simulink model "NE39bus_modified"  (R2025b)
settings: Solver=ode23tb  StartTime=0.0  StopTime=10  MaxStep=0.001  RelTol=1e-4  AbsTol=1e-6  EnableMultiTasking=on
PreLoadFcn:
  | NE39bus_data;
  | PSSMODEL=1;
  | LPSS=0;
  | WAPSS=0;
  | WAPSS2=0;
model workspace (MAT data in the model file):
  DT = 0.2
  T_EPISODE = 10
  VSG_D0 = 3
  VSG_M0 = 12
  omega_n = 314.159265359
values from neighbouring files (symbols this model uses):
  AVR_Data = [     0.01  200    0.015   10    1    1.03    -5    5 ... (first row only)    [NE39bus_data.m]    (also in NE39bus_workspace.mat = [0.01 0.01 0.01 0.01 0.01 0.01 0.01 0.01 0.01 0.01 200 200 .)
  line = [     1	2	0.0035	0.0411	0.6987	0	100	345 ... (first row only)    [NE39bus_data.m]    (also in NE39bus_modified_data.m = [     1   2   0.0035  0.0411  0.6987  0   100 345; NE39bus_workspace.mat = [1 1 2 2 2 3 3 4 4 5 6 6 ... (368 elements, 46x8)])
  mac_con = [ ... (first row only)    [NE39bus_data.m]    (also in NE39bus_workspace.mat = [1 2 3 4 5 6 7 8 9 10 39 31 ... (190 elements, 10x19)])
  MB = [1   0.2 30   1.25 40    12 160]    [NE39bus_data.m]    (also in NE39bus_modified_data.m = [1  0.2  30  1.25  40  12  160]; NE39bus_workspace.mat = [1 0.2 30 1.25 40 12 160])
  Ns = 120*60/(2)    (= 3600)    [NE39bus_data.m]    (also in NE39bus_workspace.mat)
  p0 = [1000 520.81 650 632 508 650 560 540 830 250]'./1000    [NE39bus_data.m]    (also in NE39bus_workspace.mat = [1 0.52081 0.65 0.632 0.508 0.65 0.56 0.54 0.83 0.25])
  Pn = [1 1 1 1 1 1 1 1 1 1]    [NE39bus_workspace.mat]
  s = 10    [NE39bus_data.m]    (also in NE39bus_workspace.mat)
undefined symbols (not defined in the file or in its folder): D1, Delta
libraries: spsThreePhaseVIMeasurementLib x48, spsThreePhasePISectionLineLib x34, spsGenericPowerSystemStabilizerLib x20, spsThreePhaseParallelRLCLoadLib x19, spsThreePhaseTransformerTwoWindingsLib x12, spsSynchronousMachinepuStandardLib x10, spsExcitationSystemLib x10, spsMultiBandPowerSystemStabilizerLib x10, spsSteamTurbineandGovernorLib x10, spsLoadFlowBusLib x10, spsThreePhaseProgrammableVoltageSourceLib x8, spsThreePhaseSeriesRLCBranchLib x8
(part 2 of 3)

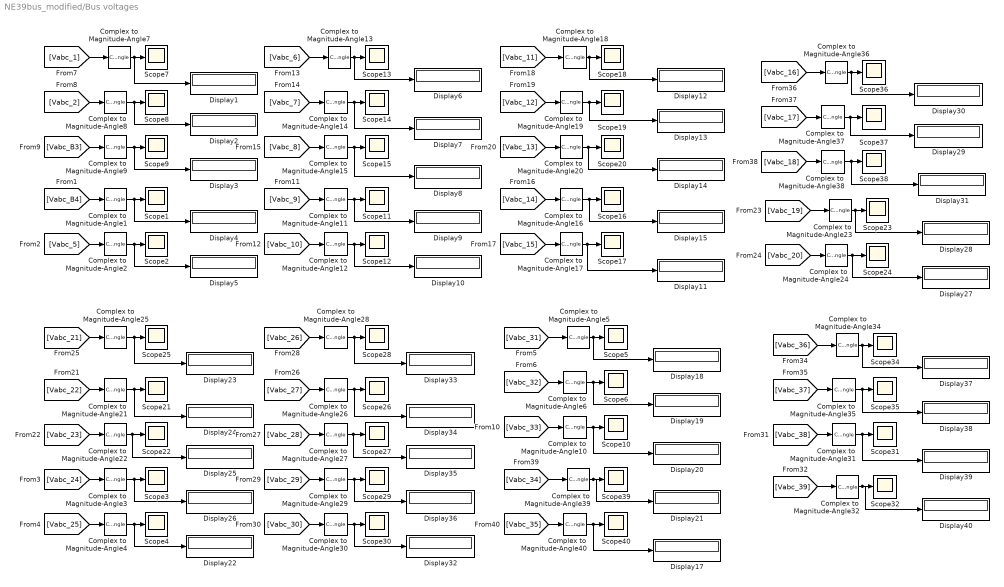
== system NE39bus_modified/Bus voltages ==
  Complex to Magnitude-Angle{1..32,34..40} (39 alike) : ComplexToMagnitudeAngle  Output=Magnitude
  Display{1..15,17..40} (39 alike) : Display
  Scope{1..32,34..40} (39 alike) : Scope
      Scope1 settings: ActiveDisplayYMinimum=-0.07  ActiveDisplayYMaximum=0.07  DataLoggingVariableName=v
      Scope10 settings: ActiveDisplayYMinimum=-0.07  ActiveDisplayYMaximum=0.07  DataLoggingVariableName=v2
      Scope11 settings: ActiveDisplayYMinimum=-0.07  ActiveDisplayYMaximum=0.07  DataLoggingVariableName=v11
      Scope12 settings: ActiveDisplayYMinimum=-0.07  ActiveDisplayYMaximum=0.07  DataLoggingVariableName=v12
      Scope13 settings: ActiveDisplayYMinimum=-0.07  ActiveDisplayYMaximum=0.07  DataLoggingVariableName=v13
      Scope14 settings: ActiveDisplayYMinimum=-0.07  ActiveDisplayYMaximum=0.07  DataLoggingVariableName=v14
      Scope15 settings: ActiveDisplayYMinimum=-0.07  ActiveDisplayYMaximum=0.07  DataLoggingVariableName=v15
      Scope16 settings: ActiveDisplayYMinimum=-0.07  ActiveDisplayYMaximum=0.07  DataLoggingVariableName=v16
      Scope17 settings: ActiveDisplayYMinimum=-0.07  ActiveDisplayYMaximum=0.07  DataLoggingVariableName=v17
      Scope18 settings: ActiveDisplayYMinimum=-0.07  ActiveDisplayYMaximum=0.07  DataLoggingVariableName=v18
      Scope19 settings: ActiveDisplayYMinimum=-0.07  ActiveDisplayYMaximum=0.07  DataLoggingVariableName=v19
      Scope2 settings: ActiveDisplayYMinimum=-0.07  ActiveDisplayYMaximum=0.07  DataLoggingVariableName=v1
      Scope20 settings: ActiveDisplayYMinimum=-0.07  ActiveDisplayYMaximum=0.07  DataLoggingVariableName=v20
      Scope21 settings: ActiveDisplayYMinimum=-0.07  ActiveDisplayYMaximum=0.07  DataLoggingVariableName=v21
      Scope22 settings: ActiveDisplayYMinimum=-0.07  ActiveDisplayYMaximum=0.07  DataLoggingVariableName=v22
      Scope23 settings: ActiveDisplayYMinimum=-0.07  ActiveDisplayYMaximum=0.07  DataLoggingVariableName=v68
      Scope24 settings: ActiveDisplayYMinimum=-0.07  ActiveDisplayYMaximum=0.07  DataLoggingVariableName=v69
      Scope25 settings: ActiveDisplayYMinimum=-0.07  ActiveDisplayYMaximum=0.07  DataLoggingVariableName=v70
      Scope26 settings: ActiveDisplayYMinimum=-0.07  ActiveDisplayYMaximum=0.07  DataLoggingVariableName=v63
      Scope27 settings: ActiveDisplayYMinimum=-0.07  ActiveDisplayYMaximum=0.07  DataLoggingVariableName=v64
      Scope28 settings: ActiveDisplayYMinimum=-0.07  ActiveDisplayYMaximum=0.07  DataLoggingVariableName=v65
      Scope29 settings: ActiveDisplayYMinimum=-0.07  ActiveDisplayYMaximum=0.07  DataLoggingVariableName=v66
      Scope3 settings: ActiveDisplayYMinimum=-0.07  ActiveDisplayYMaximum=0.07  DataLoggingVariableName=v3
      Scope30 settings: ActiveDisplayYMinimum=-0.07  ActiveDisplayYMaximum=0.07  DataLoggingVariableName=v67
      Scope31 settings: ActiveDisplayYMinimum=-0.07  ActiveDisplayYMaximum=0.07  DataLoggingVariableName=v71
      Scope32 settings: ActiveDisplayYMinimum=-0.07  ActiveDisplayYMaximum=0.07  DataLoggingVariableName=v72
      Scope34 settings: ActiveDisplayYMinimum=-0.07  ActiveDisplayYMaximum=0.07  DataLoggingVariableName=v74
      Scope35 settings: ActiveDisplayYMinimum=-0.07  ActiveDisplayYMaximum=0.07  DataLoggingVariableName=v75
      Scope36 settings: ActiveDisplayYMinimum=-0.07  ActiveDisplayYMaximum=0.07  DataLoggingVariableName=v48
      Scope37 settings: ActiveDisplayYMinimum=-0.07  ActiveDisplayYMaximum=0.07  DataLoggingVariableName=v49
      Scope38 settings: ActiveDisplayYMinimum=-0.07  ActiveDisplayYMaximum=0.07  DataLoggingVariableName=v50
      Scope39 settings: ActiveDisplayYMinimum=-0.07  ActiveDisplayYMaximum=0.07  DataLoggingVariableName=v51
      Scope4 settings: ActiveDisplayYMinimum=-0.07  ActiveDisplayYMaximum=0.07  DataLoggingVariableName=v4
      Scope40 settings: ActiveDisplayYMinimum=-0.07  ActiveDisplayYMaximum=0.07  DataLoggingVariableName=v62
      Scope5 settings: ActiveDisplayYMinimum=-0.07  ActiveDisplayYMaximum=0.07  DataLoggingVariableName=v5
      Scope6 settings: ActiveDisplayYMinimum=-0.07  ActiveDisplayYMaximum=0.07  DataLoggingVariableName=v10
      Scope7 settings: ActiveDisplayYMinimum=-0.07  ActiveDisplayYMaximum=0.07  DataLoggingVariableName=v6
      Scope8 settings: ActiveDisplayYMinimum=-0.07  ActiveDisplayYMaximum=0.07  DataLoggingVariableName=v8
      Scope9 settings: ActiveDisplayYMinimum=-0.07  ActiveDisplayYMaximum=0.07  DataLoggingVariableName=v9
  wires:
  [Vabc_1] -> Complex to Magnitude-Angle7/1
  Complex to Magnitude-Angle7/1 -> Display1/1, Scope7/1
  [Vabc_2] -> Complex to Magnitude-Angle8/1
  Complex to Magnitude-Angle8/1 -> Display2/1, Scope8/1
  [Vabc_B3] -> Complex to Magnitude-Angle9/1
  Complex to Magnitude-Angle9/1 -> Display3/1, Scope9/1
  [Vabc_B4] -> Complex to Magnitude-Angle1/1
  Complex to Magnitude-Angle1/1 -> Display4/1, Scope1/1
  [Vabc_5] -> Complex to Magnitude-Angle2/1
  Complex to Magnitude-Angle2/1 -> Display5/1, Scope2/1
  [Vabc_31] -> Complex to Magnitude-Angle5/1
  [Vabc_32] -> Complex to Magnitude-Angle6/1
  [Vabc_33] -> Complex to Magnitude-Angle10/1
  [Vabc_24] -> Complex to Magnitude-Angle3/1
  [Vabc_25] -> Complex to Magnitude-Angle4/1
  [Vabc_6] -> Complex to Magnitude-Angle13/1
  [Vabc_7] -> Complex to Magnitude-Angle14/1
  [Vabc_8] -> Complex to Magnitude-Angle15/1
  [Vabc_9] -> Complex to Magnitude-Angle11/1
  [Vabc_10] -> Complex to Magnitude-Angle12/1
  [Vabc_11] -> Complex to Magnitude-Angle18/1
  Complex to Magnitude-Angle18/1 -> Display12/1, Scope18/1
  [Vabc_12] -> Complex to Magnitude-Angle19/1
  [Vabc_13] -> Complex to Magnitude-Angle20/1
  Complex to Magnitude-Angle20/1 -> Display14/1, Scope20/1
  [Vabc_14] -> Complex to Magnitude-Angle16/1
  Complex to Magnitude-Angle16/1 -> Display15/1, Scope16/1
  [Vabc_15] -> Complex to Magnitude-Angle17/1
  Complex to Magnitude-Angle17/1 -> Display11/1, Scope17/1
  [Vabc_19] -> Complex to Magnitude-Angle23/1
  [Vabc_20] -> Complex to Magnitude-Angle24/1
  [Vabc_21] -> Complex to Magnitude-Angle25/1
  [Vabc_22] -> Complex to Magnitude-Angle21/1
  [Vabc_23] -> Complex to Magnitude-Angle22/1
  Complex to Magnitude-Angle13/1 -> Display6/1, Scope13/1
  Complex to Magnitude-Angle14/1 -> Display7/1, Scope14/1
  Complex to Magnitude-Angle15/1 -> Display8/1, Scope15/1
  Complex to Magnitude-Angle11/1 -> Display9/1, Scope11/1
  Complex to Magnitude-Angle12/1 -> Display10/1, Scope12/1
  Complex to Magnitude-Angle19/1 -> Display13/1, Scope19/1
  [Vabc_16] -> Complex to Magnitude-Angle36/1
  [Vabc_17] -> Complex to Magnitude-Angle37/1
  [Vabc_18] -> Complex to Magnitude-Angle38/1
  Complex to Magnitude-Angle38/1 -> Display31/1, Scope38/1
  [Vabc_34] -> Complex to Magnitude-Angle39/1
  [Vabc_35] -> Complex to Magnitude-Angle40/1
  Complex to Magnitude-Angle5/1 -> Display18/1, Scope5/1
  Complex to Magnitude-Angle10/1 -> Display20/1, Scope10/1
  Complex to Magnitude-Angle39/1 -> Display21/1, Scope39/1
  Complex to Magnitude-Angle40/1 -> Display17/1, Scope40/1
  Complex to Magnitude-Angle6/1 -> Display19/1, Scope6/1
  Complex to Magnitude-Angle25/1 -> Display23/1, Scope25/1
  Complex to Magnitude-Angle22/1 -> Display25/1, Scope22/1
  Complex to Magnitude-Angle3/1 -> Display26/1, Scope3/1
  Complex to Magnitude-Angle4/1 -> Display22/1, Scope4/1
  Complex to Magnitude-Angle21/1 -> Display24/1, Scope21/1
  Complex to Magnitude-Angle23/1 -> Display28/1, Scope23/1
  Complex to Magnitude-Angle24/1 -> Display27/1, Scope24/1
  Complex to Magnitude-Angle36/1 -> Display30/1, Scope36/1
  Complex to Magnitude-Angle37/1 -> Display29/1, Scope37/1
  [Vabc_29] -> Complex to Magnitude-Angle29/1
  [Vabc_30] -> Complex to Magnitude-Angle30/1
  [Vabc_26] -> Complex to Magnitude-Angle28/1
  [Vabc_27] -> Complex to Magnitude-Angle26/1
  [Vabc_28] -> Complex to Magnitude-Angle27/1
  Complex to Magnitude-Angle28/1 -> Display33/1, Scope28/1
  Complex to Magnitude-Angle27/1 -> Display35/1, Scope27/1
  Complex to Magnitude-Angle29/1 -> Display36/1, Scope29/1
  Complex to Magnitude-Angle30/1 -> Display32/1, Scope30/1
  Complex to Magnitude-Angle26/1 -> Display34/1, Scope26/1
  [Vabc_36] -> Complex to Magnitude-Angle34/1
  [Vabc_37] -> Complex to Magnitude-Angle35/1
  [Vabc_38] -> Complex to Magnitude-Angle31/1
  [Vabc_39] -> Complex to Magnitude-Angle32/1
  Complex to Magnitude-Angle34/1 -> Display37/1, Scope34/1
  Complex to Magnitude-Angle31/1 -> Display39/1, Scope31/1
  Complex to Magnitude-Angle32/1 -> Display40/1, Scope32/1
  Complex to Magnitude-Angle35/1 -> Display38/1, Scope35/1

== system NE39bus_modified/G1 ==
  G1 : spsSynchronousMachinepuStandardLib/Synchronous Machine pu Standard  PresetModel=No  MechanicalLoad=Mechanical power Pm  ShowDetailedParameters=on  RotorType=Round  Units=per unit standard parameters  MeasurementBus=off  NominalParameters="[Pn(1,1)*1E9  345000   60 ]"  Reactances1="[mac_con(1,6:8)  mac_con(1,11:13)  mac_con(1,4)]"  Reactances2=[ 1.305, 0.296, 0.252, 0.474, 0.243, 0.18 ]  dAxisTimeConstants=Open-circuit  qAxisTimeConstants=Open-circuit  TimeConstants1=[]  TimeConstants2="[mac_con(1,9:10)  mac_con(1,14:15)]"  TimeConstants3=[]  TimeConstants4=[]  TimeConstants5=[ 1.01, 0.053, 0.1 ]  TimeConstants6=[]  TimeConstants7=[]  TimeConstants8=[]  StatorResistance=mac_con(1,5)  Mechanical="[ mac_con(1,16)  0  4]"  PolePairs=4  InitialConditions=[0 -53.3817 1.03438 1.03438 1.03438 11.5505 -108.45 131.55 1.07168]  SetSaturation=off  Saturation=[0.6404,0.7127,0.8441,0.9214,0.9956,1.082,1.19,1.316,1.457;0.7,0.7698,0.8872,0.9466,0.9969,1.046,1.1,1.151,1.201]  LoadFlowParameters=[1 1000000000 0 0 0]  TsPowergui=0  TsBlock=-1  IterativeModel=Forward Euler  IterativeDiscreteModel=Trapezoidal non iterative  BusType=PV  Pref=p0(1,1)*1E9  Qref=0  Qmin=-inf  Qmax=inf  PLF=0  QLF=0
  M1: Turbine & Regulators : Subsystem
  Pref1 : Constant
  Vref1 : Constant
  A : PMIOPort  Side=Left
  B : PMIOPort  Port=2  Side=Left
  C : PMIOPort  Port=3  Side=Left
  wires:
  Pref1/1 -> M1: Turbine & Regulators/2(Pref1)
  [PSSmodel] -> M1: Turbine & Regulators/4(PSS1)
  M1: Turbine & Regulators/1(Pm1) -> G1/1
  M1: Turbine & Regulators/2(Vf1) -> G1/2
  G1/1 -> M1: Turbine & Regulators/1(m)
  Vref1/1 -> M1: Turbine & Regulators/3(Vref1)
  connections:
  A/RConn1 -- G1/RConn1
  B/RConn1 -- G1/RConn2
  C/RConn1 -- G1/RConn3

== system NE39bus_modified/G10 ==
  G10 : spsSynchronousMachinepuStandardLib/Synchronous Machine pu Standard  PresetModel=No  MechanicalLoad=Mechanical power Pm  ShowDetailedParameters=on  RotorType=Round  Units=per unit standard parameters  MeasurementBus=off  NominalParameters="[Pn(10,1)*1E9  22000   60 ]"  Reactances1="[mac_con(10,6:8)  mac_con(10,11:13)  mac_con(10,4)]"  Reactances2=[ 1.305, 0.296, 0.252, 0.474, 0.243, 0.18 ]  dAxisTimeConstants=Open-circuit  qAxisTimeConstants=Open-circuit  TimeConstants1=[]  TimeConstants2="[mac_con(10,9:10)  mac_con(10,14:15)]"  TimeConstants3=[]  TimeConstants4=[]  TimeConstants5=[ 1.01, 0.053, 0.1 ]  TimeConstants6=[]  TimeConstants7=[]  TimeConstants8=[]  StatorResistance=mac_con(10,5)  Mechanical="[ mac_con(10,16)  0  4]"  PolePairs=4  InitialConditions=[0 -76.9944 0.265611 0.265611 0.265611 -15.9627 -135.963 104.037 1.1157]  SetSaturation=off  Saturation=[0.6404,0.7127,0.8441,0.9214,0.9956,1.082,1.19,1.316,1.457;0.7,0.7698,0.8872,0.9466,0.9969,1.046,1.1,1.151,1.201]  LoadFlowParameters=[1 250000000 0 0 0]  TsPowergui=0  TsBlock=-1  IterativeModel=Forward Euler  IterativeDiscreteModel=Trapezoidal non iterative  BusType=PV  Pref=p0(10,1)*1E9  Qref=0  Qmin=-inf  Qmax=inf  PLF=0  QLF=0
  M10: Turbine & Regulators : Subsystem
  Pref10 : Constant  Value=0.25
  Vref10 : Constant
  A : PMIOPort  Side=Left
  B : PMIOPort  Port=2  Side=Left
  C : PMIOPort  Port=3  Side=Left
  wires:
  Pref10/1 -> M10: Turbine & Regulators/2(Pref10)
  [PSSmodel] -> M10: Turbine & Regulators/4(PSS10)
  M10: Turbine & Regulators/1(Pm10) -> G10/1
  M10: Turbine & Regulators/2(Vf10) -> G10/2
  G10/1 -> M10: Turbine & Regulators/1(m)
  Vref10/1 -> M10: Turbine & Regulators/3(Vref10)
  connections:
  A/RConn1 -- G10/RConn1
  B/RConn1 -- G10/RConn2
  C/RConn1 -- G10/RConn3

== system NE39bus_modified/G2 ==
  G2 : spsSynchronousMachinepuStandardLib/Synchronous Machine pu Standard  PresetModel=No  MechanicalLoad=Mechanical power Pm  ShowDetailedParameters=on  RotorType=Round  Units=per unit standard parameters  MeasurementBus=off  NominalParameters="[Pn(2,1)*1E9  22000   60 ]"  Reactances1="[mac_con(2,6:8)  mac_con(2,11:13)  mac_con(2,4)]"  Reactances2=[ 1.305, 0.296, 0.252, 0.474, 0.243, 0.18 ]  dAxisTimeConstants=Open-circuit  qAxisTimeConstants=Open-circuit  TimeConstants1=[]  TimeConstants2="[mac_con(2,9:10)  mac_con(2,14:15)]"  TimeConstants3=[]  TimeConstants4=[]  TimeConstants5=[ 1.01, 0.053, 0.1 ]  TimeConstants6=[]  TimeConstants7=[]  TimeConstants8=[]  StatorResistance=mac_con(2,5)  Mechanical="[ mac_con(2,16)  0  4]"  PolePairs=4  InitialConditions=[0 -63.2657 0.339533 0.339533 0.339533 -35.2425 -155.242 84.7575 1.77729]  SetSaturation=off  Saturation=[0.6404,0.7127,0.8441,0.9214,0.9956,1.082,1.19,1.316,1.457;0.7,0.7698,0.8872,0.9466,0.9969,1.046,1.1,1.151,1.201]  LoadFlowParameters=[2 546000000 0 0 0]  TsPowergui=0  TsBlock=-1  IterativeModel=Forward Euler  IterativeDiscreteModel=Trapezoidal non iterative  BusType=swing  Pref=0  Qref=0  Qmin=-inf  Qmax=inf  PLF=0  QLF=0
  M2: Turbine & Regulators : Subsystem
  Pref2 : Constant  Value=0.277303
  Vref2 : Constant
  A : PMIOPort  Side=Left
  B : PMIOPort  Port=2  Side=Left
  C : PMIOPort  Port=3  Side=Left
  wires:
  Pref2/1 -> M2: Turbine & Regulators/2(Pref2)
  [PSSmodel] -> M2: Turbine & Regulators/4(PSS2)
  M2: Turbine & Regulators/1(Pm2) -> G2/1
  M2: Turbine & Regulators/2(Vf2) -> G2/2
  G2/1 -> M2: Turbine & Regulators/1(m2)
  Vref2/1 -> M2: Turbine & Regulators/3(Vref2)
  connections:
  G2/RConn1 -- A/RConn1
  B/RConn1 -- G2/RConn2
  C/RConn1 -- G2/RConn3

== system NE39bus_modified/G3 ==
  G3 : spsSynchronousMachinepuStandardLib/Synchronous Machine pu Standard  PresetModel=No  MechanicalLoad=Mechanical power Pm  ShowDetailedParameters=on  RotorType=Round  Units=per unit standard parameters  MeasurementBus=off  NominalParameters="[Pn(3,1)*1E9  22000   60 ]"  Reactances1="[mac_con(3,6:8)  mac_con(3,11:13)  mac_con(3,4)]"  Reactances2=[ 1.305, 0.296, 0.252, 0.474, 0.243, 0.18 ]  dAxisTimeConstants=Open-circuit  qAxisTimeConstants=Open-circuit  TimeConstants1=[]  TimeConstants2="[mac_con(3,9:10)  mac_con(3,14:15)]"  TimeConstants3=[]  TimeConstants4=[]  TimeConstants5=[ 1.01, 0.053, 0.1 ]  TimeConstants6=[]  TimeConstants7=[]  TimeConstants8=[]  StatorResistance=mac_con(3,5)  Mechanical="[ mac_con(3,16)  0  4]"  PolePairs=4  InitialConditions=[0 -37.958 0.689466 0.689466 0.689466 -12.356 -132.356 107.644 2.25944]  SetSaturation=off  Saturation=[0.6404,0.7127,0.8441,0.9214,0.9956,1.082,1.19,1.316,1.457;0.7,0.7698,0.8872,0.9466,0.9969,1.046,1.1,1.151,1.201]  LoadFlowParameters=[1 650000000 0 0 0]  TsPowergui=0  TsBlock=-1  IterativeModel=Forward Euler  IterativeDiscreteModel=Trapezoidal non iterative  BusType=PV  Pref=p0(3,1)*1E9  Qref=0  Qmin=-inf  Qmax=inf  PLF=0  QLF=0
  M3: Turbine & Regulators : Subsystem
  Pref3 : Constant  Value=0.65
  Vref3 : Constant
  A : PMIOPort  Side=Left
  B : PMIOPort  Port=2  Side=Left
  C : PMIOPort  Port=3  Side=Left
  wires:
  Pref3/1 -> M3: Turbine & Regulators/2(Pref3)
  G3/1 -> M3: Turbine & Regulators/1(m3)
  M3: Turbine & Regulators/1(Pm3) -> G3/1
  M3: Turbine & Regulators/2(Vf3) -> G3/2
  Vref3/1 -> M3: Turbine & Regulators/3(Vref3)
  [PSSmodel] -> M3: Turbine & Regulators/4(PSS3)
  connections:
  A/RConn1 -- G3/RConn1
  B/RConn1 -- G3/RConn2
  C/RConn1 -- G3/RConn3

== system NE39bus_modified/G4 ==
  G4 : spsSynchronousMachinepuStandardLib/Synchronous Machine pu Standard  PresetModel=No  MechanicalLoad=Mechanical power Pm  ShowDetailedParameters=on  RotorType=Round  Units=per unit standard parameters  MeasurementBus=off  NominalParameters="[Pn(4,1)*1E9  22000   60 ]"  Reactances1="[mac_con(4,6:8)  mac_con(4,11:13)  mac_con(4,4)]"  Reactances2=[ 1.305, 0.296, 0.252, 0.474, 0.243, 0.18 ]  dAxisTimeConstants=Open-circuit  qAxisTimeConstants=Open-circuit  TimeConstants1=[]  TimeConstants2="[mac_con(4,9:10)  mac_con(4,14:15)]"  TimeConstants3=[]  TimeConstants4=[]  TimeConstants5=[ 1.01, 0.053, 0.1 ]  TimeConstants6=[]  TimeConstants7=[]  TimeConstants8=[]  StatorResistance=mac_con(4,5)  Mechanical="[ mac_con(4,16)  0  4]"  PolePairs=4  InitialConditions=[0 -27.7466 0.647548 0.647548 0.647548 -0.416201 -120.416 119.584 2.14879]  SetSaturation=off  Saturation=[0.6404,0.7127,0.8441,0.9214,0.9956,1.082,1.19,1.316,1.457;0.7,0.7698,0.8872,0.9466,0.9969,1.046,1.1,1.151,1.201]  LoadFlowParameters=[1 632000000 22000 0 0]  TsPowergui=0  TsBlock=-1  IterativeModel=Forward Euler  IterativeDiscreteModel=Trapezoidal non iterative  BusType=PV  Pref=p0(4,1)*1E9  Qref=0  Qmin=-inf  Qmax=inf  PLF=0  QLF=0
  M4: Turbine & Regulators : Subsystem
  Pref4 : Constant  Value=0.632
  Vref4 : Constant
  A : PMIOPort  Side=Left
  B : PMIOPort  Port=2  Side=Left
  C : PMIOPort  Port=3  Side=Left
  wires:
  G4/1 -> M4: Turbine & Regulators/1(m4)
  Pref4/1 -> M4: Turbine & Regulators/2(Pref4)
  Vref4/1 -> M4: Turbine & Regulators/3(Vref4)
  [PSSmodel] -> M4: Turbine & Regulators/4(PSS4)
  M4: Turbine & Regulators/1(Pm4) -> G4/1
  M4: Turbine & Regulators/2(Vf4) -> G4/2
  connections:
  A/RConn1 -- G4/RConn1
  B/RConn1 -- G4/RConn2
  C/RConn1 -- G4/RConn3

== system NE39bus_modified/G5 ==
  G5 : spsSynchronousMachinepuStandardLib/Synchronous Machine pu Standard  PresetModel=No  MechanicalLoad=Mechanical power Pm  ShowDetailedParameters=on  RotorType=Round  Units=per unit standard parameters  MeasurementBus=off  NominalParameters="[Pn(5,1)*1E9  22000   60 ]"  Reactances1="[mac_con(5,6:8)  mac_con(5,11:13)  mac_con(5,4)]"  Reactances2=[ 1.305, 0.296, 0.252, 0.474, 0.243, 0.18 ]  dAxisTimeConstants=Open-circuit  qAxisTimeConstants=Open-circuit  TimeConstants1=[]  TimeConstants2="[mac_con(5,9:10)  mac_con(5,14:15)]"  TimeConstants3=[]  TimeConstants4=[]  TimeConstants5=[ 1.01, 0.053, 0.1 ]  TimeConstants6=[]  TimeConstants7=[]  TimeConstants8=[]  StatorResistance=mac_con(5,5)  Mechanical="[ mac_con(5,16)  0  4]"  PolePairs=4  InitialConditions=[0 -18.657 0.524928 0.524928 0.524928 -3.22796 -123.228 116.772 3.89055]  SetSaturation=off  Saturation=[0.6404,0.7127,0.8441,0.9214,0.9956,1.082,1.19,1.316,1.457;0.7,0.7698,0.8872,0.9466,0.9969,1.046,1.1,1.151,1.201]  LoadFlowParameters=[1 508000000 0 0 0]  TsPowergui=0  TsBlock=-1  IterativeModel=Forward Euler  IterativeDiscreteModel=Trapezoidal non iterative  BusType=PV  Pref=p0(5,1)*1E9  Qref=0  Qmin=-inf  Qmax=inf  PLF=0  QLF=0
  M5: Turbine & Regulators : Subsystem
  Pref5 : Constant  Value=0.508
  Vref5 : Constant
  A : PMIOPort  Side=Left
  B : PMIOPort  Port=2  Side=Left
  C : PMIOPort  Port=3  Side=Left
  wires:
  G5/1 -> M5: Turbine & Regulators/1(m5)
  M5: Turbine & Regulators/2(Vf5) -> G5/2
  M5: Turbine & Regulators/1(Pm5) -> G5/1
  Pref5/1 -> M5: Turbine & Regulators/2(Pref5)
  Vref5/1 -> M5: Turbine & Regulators/3(Vref5)
  [PSSmodel] -> M5: Turbine & Regulators/4(PSS5)
  connections:
  G5/RConn1 -- A/RConn1
  G5/RConn2 -- B/RConn1
  G5/RConn3 -- C/RConn1

== system NE39bus_modified/G6 ==
  G6 : spsSynchronousMachinepuStandardLib/Synchronous Machine pu Standard  PresetModel=No  MechanicalLoad=Mechanical power Pm  ShowDetailedParameters=on  RotorType=Round  Units=per unit standard parameters  MeasurementBus=off  NominalParameters="[Pn(6,1)*1E9  22000   60 ]"  Reactances1="[mac_con(6,6:8)  mac_con(6,11:13)  mac_con(6,4)]"  Reactances2=[ 1.305, 0.296, 0.252, 0.474, 0.243, 0.18 ]  dAxisTimeConstants=Open-circuit  qAxisTimeConstants=Open-circuit  TimeConstants1=[]  TimeConstants2="[mac_con(6,9:10)  mac_con(6,14:15)]"  TimeConstants3=[]  TimeConstants4=[]  TimeConstants5=[ 1.01, 0.053, 0.1 ]  TimeConstants6=[]  TimeConstants7=[]  TimeConstants8=[]  StatorResistance=mac_con(6,5)  Mechanical="[ mac_con(6,16)  0  4]"  PolePairs=4  InitialConditions=[0 -28.3893 0.677322 0.677322 0.677322 -1.75458 -121.755 118.245 2.21937]  SetSaturation=off  Saturation=[0.6404,0.7127,0.8441,0.9214,0.9956,1.082,1.19,1.316,1.457;0.7,0.7698,0.8872,0.9466,0.9969,1.046,1.1,1.151,1.201]  LoadFlowParameters=[1 650000000 0 0 0]  TsPowergui=0  TsBlock=-1  IterativeModel=Forward Euler  IterativeDiscreteModel=Trapezoidal non iterative  BusType=PV  Pref=p0(6,1)*1E9  Qref=0  Qmin=-inf  Qmax=inf  PLF=0  QLF=0
  M6: Turbine & Regulators : Subsystem
  Pref6 : Constant  Value=0.65
  Vref6 : Constant
  A : PMIOPort  Side=Left
  B : PMIOPort  Port=2  Side=Left
  C : PMIOPort  Port=3  Side=Left
  wires:
  M6: Turbine & Regulators/1(Pm6) -> G6/1
  G6/1 -> M6: Turbine & Regulators/1(m6)
  Vref6/1 -> M6: Turbine & Regulators/3(Vref6)
  Pref6/1 -> M6: Turbine & Regulators/2(Pref6)
  [PSSmodel] -> M6: Turbine & Regulators/4(PSS6)
  M6: Turbine & Regulators/2(Vf6) -> G6/2
  connections:
  A/RConn1 -- G6/RConn1
  B/RConn1 -- G6/RConn2
  C/RConn1 -- G6/RConn3

== system NE39bus_modified/G7 ==
  G7 : spsSynchronousMachinepuStandardLib/Synchronous Machine pu Standard  PresetModel=No  MechanicalLoad=Mechanical power Pm  ShowDetailedParameters=on  RotorType=Round  Units=per unit standard parameters  MeasurementBus=off  NominalParameters="[Pn(7,1)*1E9  22000   60 ]"  Reactances1="[mac_con(7,6:8)  mac_con(7,11:13)  mac_con(7,4)]"  Reactances2=[ 1.305, 0.296, 0.252, 0.474, 0.243, 0.18 ]  dAxisTimeConstants=Open-circuit  qAxisTimeConstants=Open-circuit  TimeConstants1=[]  TimeConstants2="[mac_con(7,9:10)  mac_con(7,14:15)]"  TimeConstants3=[]  TimeConstants4=[]  TimeConstants5=[ 1.01, 0.053, 0.1 ]  TimeConstants6=[]  TimeConstants7=[]  TimeConstants8=[]  StatorResistance=mac_con(7,5)  Mechanical="[ mac_con(7,16)  0  4]"  PolePairs=4  InitialConditions=[0 -22.3007 0.574969 0.574969 0.574969 4.77124 -115.229 124.771 2.15543]  SetSaturation=off  Saturation=[0.6404,0.7127,0.8441,0.9214,0.9956,1.082,1.19,1.316,1.457;0.7,0.7698,0.8872,0.9466,0.9969,1.046,1.1,1.151,1.201]  LoadFlowParameters=[1 560000000 0 0 0]  TsPowergui=0  TsBlock=-1  IterativeModel=Forward Euler  IterativeDiscreteModel=Trapezoidal non iterative  BusType=PV  Pref=p0(7,1)*1E9  Qref=0  Qmin=-inf  Qmax=inf  PLF=0  QLF=0
  M7: Turbine & Regulators : Subsystem
  Pref7 : Constant  Value=0.56
  Vref7 : Constant
  A : PMIOPort  Side=Left
  B : PMIOPort  Port=2  Side=Left
  C : PMIOPort  Port=3  Side=Left
  wires:
  M7: Turbine & Regulators/1(Pm7) -> G7/1
  M7: Turbine & Regulators/2(Vf7) -> G7/2
  G7/1 -> M7: Turbine & Regulators/1(m7)
  Pref7/1 -> M7: Turbine & Regulators/2(Pref7)
  Vref7/1 -> M7: Turbine & Regulators/3(Vref7)
  [PSSmodel] -> M7: Turbine & Regulators/4(PSS7)
  connections:
  G7/RConn1 -- A/RConn1
  G7/RConn2 -- B/RConn1
  G7/RConn3 -- C/RConn1

== system NE39bus_modified/G8 ==
  G8 : spsSynchronousMachinepuStandardLib/Synchronous Machine pu Standard  PresetModel=No  MechanicalLoad=Mechanical power Pm  ShowDetailedParameters=on  RotorType=Round  Units=per unit standard parameters  MeasurementBus=off  NominalParameters="[Pn(8,1)*1e9  22000   60 ]"  Reactances1="[mac_con(8,6:8)  mac_con(8,11:13)  mac_con(8,4)]"  Reactances2=[ 1.305, 0.296, 0.252, 0.474, 0.243, 0.18 ]  dAxisTimeConstants=Open-circuit  qAxisTimeConstants=Open-circuit  TimeConstants1=[]  TimeConstants2="[mac_con(8,9:10)  mac_con(8,14:15)]"  TimeConstants3=[]  TimeConstants4=[]  TimeConstants5=[ 1.01, 0.053, 0.1 ]  TimeConstants6=[]  TimeConstants7=[]  TimeConstants8=[]  StatorResistance=mac_con(8,5)  Mechanical="[ mac_con(8,16)  0  4]"  PolePairs=4  InitialConditions=[0 -25.6939 0.5409 0.5409 0.5409 6.7214 -113.279 126.721 1.90805]  SetSaturation=off  Saturation=[0.6404,0.7127,0.8441,0.9214,0.9956,1.082,1.19,1.316,1.457;0.7,0.7698,0.8872,0.9466,0.9969,1.046,1.1,1.151,1.201]  LoadFlowParameters=[1 540000000 0 0 0]  TsPowergui=0  TsBlock=-1  IterativeModel=Forward Euler  IterativeDiscreteModel=Trapezoidal non iterative  BusType=PV  Pref=p0(8,1)*1E9  Qref=0  Qmin=-inf  Qmax=inf  PLF=0  QLF=0
  M8: Turbine & Regulators : Subsystem
  Pref8 : Constant  Value=0.54
  Vref8 : Constant
  A : PMIOPort  Side=Left
  B : PMIOPort  Port=2  Side=Left
  C : PMIOPort  Port=3  Side=Left
  wires:
  M8: Turbine & Regulators/1(Pm8) -> G8/1
  M8: Turbine & Regulators/2(Vf8) -> G8/2
  G8/1 -> M8: Turbine & Regulators/1(m8)
  Vref8/1 -> M8: Turbine & Regulators/3(Vref8)
  [PSSmodel] -> M8: Turbine & Regulators/4(PSS8)
  Pref8/1 -> M8: Turbine & Regulators/2(Pref8)
  connections:
  A/RConn1 -- G8/RConn1
  B/RConn1 -- G8/RConn2
  C/RConn1 -- G8/RConn3

== system NE39bus_modified/G9 ==
  G9 : spsSynchronousMachinepuStandardLib/Synchronous Machine pu Standard  PresetModel=No  MechanicalLoad=Mechanical power Pm  ShowDetailedParameters=on  RotorType=Round  Units=per unit standard parameters  MeasurementBus=off  NominalParameters="[Pn(9,1)*1E9  22000   60 ]"  Reactances1="[mac_con(9,6:8)  mac_con(9,11:13)  mac_con(9,4)]"  Reactances2=[ 1.305, 0.296, 0.252, 0.474, 0.243, 0.18 ]  dAxisTimeConstants=Open-circuit  qAxisTimeConstants=Open-circuit  TimeConstants1=[]  TimeConstants2="[mac_con(9,9:10)  mac_con(9,14:15)]"  TimeConstants3=[]  TimeConstants4=[]  TimeConstants5=[ 1.01, 0.053, 0.1 ]  TimeConstants6=[]  TimeConstants7=[]  TimeConstants8=[]  StatorResistance=mac_con(9,5)  Mechanical="[ mac_con(9,16)  0  4]"  PolePairs=4  InitialConditions=[0 -16.7125 0.832308 0.832308 0.832308 12.5378 -107.462 132.538 2.08155]  SetSaturation=off  Saturation=[0.6404,0.7127,0.8441,0.9214,0.9956,1.082,1.19,1.316,1.457;0.7,0.7698,0.8872,0.9466,0.9969,1.046,1.1,1.151,1.201]  LoadFlowParameters=[1 830000000 0 0 0]  TsPowergui=0  TsBlock=-1  IterativeModel=Forward Euler  IterativeDiscreteModel=Trapezoidal non iterative  BusType=PV  Pref=p0(9,1)*1E9  Qref=0  Qmin=-inf  Qmax=inf  PLF=0  QLF=0
  "M9: Turbine & Regulators " : Subsystem
  Pref9 : Constant  Value=0.83
  Vref9 : Constant
  A : PMIOPort  Side=Left
  B : PMIOPort  Port=2  Side=Left
  C : PMIOPort  Port=3  Side=Left
  wires:
  Pref9/1 -> "M9: Turbine & Regulators "/2(Pref9)
  "M9: Turbine & Regulators "/1(Pm9) -> G9/1
  "M9: Turbine & Regulators "/2(Vf9) -> G9/2
  G9/1 -> "M9: Turbine & Regulators "/1(m9)
  [PSSmodel] -> "M9: Turbine & Regulators "/4(PSS9)
  Vref9/1 -> "M9: Turbine & Regulators "/3(Vref9)
  connections:
  A/RConn1 -- G9/RConn1
  B/RConn1 -- G9/RConn2
  C/RConn1 -- G9/RConn3

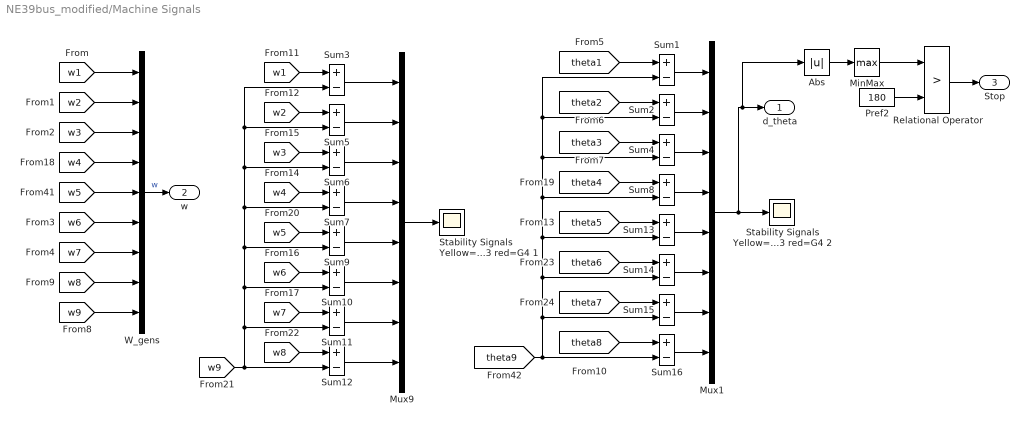
== system NE39bus_modified/Machine Signals ==
  Abs : Abs
  MinMax : MinMax  Function=max  InputSameDT=on  SaturateOnIntegerOverflow=on
  Mux1 : Mux  Inputs=8
  Mux9 : Mux  Inputs=8
  Pref2 : Constant  Value=180
  Relational Operator : RelationalOperator  Operator=>
  Stability Signals Yellow=G1 mag=G2 cyan=G3 red=G4 1 : Scope
      settings: Title=PSS  ActiveDisplayYMinimum=-0.15  ActiveDisplayYMaximum=0.15
  Stability Signals Yellow=G1 mag=G2 cyan=G3 red=G4 2 : Scope
      settings: Title=PSS  ActiveDisplayYMinimum=-0.15  ActiveDisplayYMaximum=0.15
  Sum{1..16} (16 alike) : Sum  Inputs=+-  InputSameDT=on  SaturateOnIntegerOverflow=on  OutDataTypeStr=Inherit: Same as first input
  W_gens : Mux  Inputs=9
  d_theta : Outport
  w : Outport  Port=2
  Stop : Outport  Port=3
  wires:
  Abs/1 -> MinMax/1
  Pref2/1 -> Relational Operator/2
  MinMax/1 -> Relational Operator/1
  W_gens/1 -> w/1  "w"
  Relational Operator/1 -> Stop/1
  Mux9/1 -> Stability Signals Yellow=G1 mag=G2 cyan=G3 red=G4 1/1
  [w1] -> W_gens/1
  [w2] -> W_gens/2
  [w4] -> W_gens/4
  [w3] -> W_gens/3
  [w5] -> W_gens/5
  [w9] -> W_gens/9
  [w8] -> W_gens/8
  [w7] -> W_gens/7
  [w6] -> W_gens/6
  [w1] -> Sum3/1
  [w2] -> Sum5/1
  [w4] -> Sum7/1
  [w3] -> Sum6/1
  [w5] -> Sum9/1
  [w9] -> Sum11/2, Sum10/2, Sum9/2, Sum7/2, Sum6/2, Sum5/2, Sum3/2, Sum12/2
  [w8] -> Sum12/1
  [w7] -> Sum11/1
  [w6] -> Sum10/1
  Sum7/1 -> Mux9/4
  Sum6/1 -> Mux9/3
  Sum5/1 -> Mux9/2
  Sum3/1 -> Mux9/1
  Sum10/1 -> Mux9/6
  Sum9/1 -> Mux9/5
  Sum11/1 -> Mux9/7
  Sum12/1 -> Mux9/8
  [theta9] -> Sum15/2, Sum14/2, Sum4/2, Sum1/2, Sum2/2, Sum8/2, Sum13/2, Sum16/2
  [theta8] -> Sum16/1
  [theta1] -> Sum1/1
  [theta2] -> Sum2/1
  [theta3] -> Sum4/1
  [theta4] -> Sum8/1
  [theta5] -> Sum13/1
  [theta6] -> Sum14/1
  [theta7] -> Sum15/1
  Sum2/1 -> Mux1/2
  Sum1/1 -> Mux1/1
  Sum4/1 -> Mux1/3
  Sum8/1 -> Mux1/4
  Sum13/1 -> Mux1/5
  Sum14/1 -> Mux1/6
  Sum15/1 -> Mux1/7
  Sum16/1 -> Mux1/8
  Mux1/1 -> Abs/1, d_theta/1, Stability Signals Yellow=G1 mag=G2 cyan=G3 red=G4 2/1

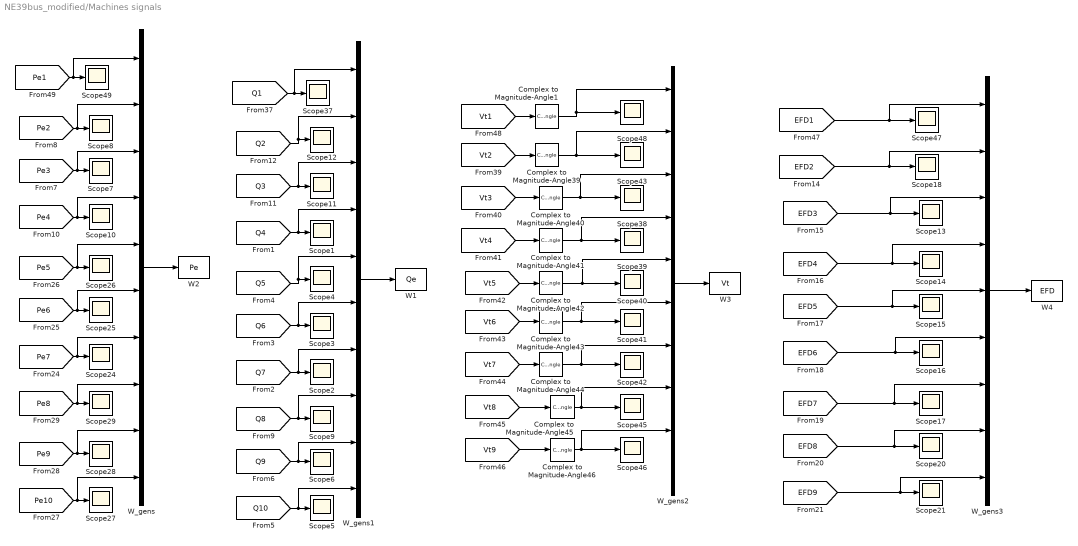
== system NE39bus_modified/Machines signals ==
  Complex to Magnitude-Angle{1,39..46} (9 alike) : ComplexToMagnitudeAngle  Output=Magnitude
  Scope{1..18,20..21,24..29,37..43,45..49} (38 alike) : Scope
      Scope1 settings: ActiveDisplayYMinimum=-0.07  ActiveDisplayYMaximum=0.07  DataLoggingVariableName=v23
      Scope10 settings: ActiveDisplayYMinimum=-0.07  ActiveDisplayYMaximum=0.07  DataLoggingVariableName=v27
      Scope11 settings: ActiveDisplayYMinimum=-0.07  ActiveDisplayYMaximum=0.07  DataLoggingVariableName=v24
      Scope12 settings: ActiveDisplayYMinimum=-0.07  ActiveDisplayYMaximum=0.07  DataLoggingVariableName=v25
      Scope13 settings: ActiveDisplayYMinimum=-0.07  ActiveDisplayYMaximum=0.07  DataLoggingVariableName=v39
      Scope14 settings: ActiveDisplayYMinimum=-0.07  ActiveDisplayYMaximum=0.07  DataLoggingVariableName=v40
      Scope15 settings: ActiveDisplayYMinimum=-0.07  ActiveDisplayYMaximum=0.07  DataLoggingVariableName=v41
      Scope16 settings: ActiveDisplayYMinimum=-0.07  ActiveDisplayYMaximum=0.07  DataLoggingVariableName=v42
      Scope17 settings: ActiveDisplayYMinimum=-0.07  ActiveDisplayYMaximum=0.07  DataLoggingVariableName=v43
      Scope18 settings: ActiveDisplayYMinimum=-0.07  ActiveDisplayYMaximum=0.07  DataLoggingVariableName=v44
      Scope2 settings: ActiveDisplayYMinimum=-0.07  ActiveDisplayYMaximum=0.07  DataLoggingVariableName=v33
      Scope20 settings: ActiveDisplayYMinimum=-0.07  ActiveDisplayYMaximum=0.07  DataLoggingVariableName=v45
      Scope21 settings: ActiveDisplayYMinimum=-0.07  ActiveDisplayYMaximum=0.07  DataLoggingVariableName=v46
      Scope24 settings: ActiveDisplayYMinimum=-0.07  ActiveDisplayYMaximum=0.07  DataLoggingVariableName=v28
      Scope25 settings: ActiveDisplayYMinimum=-0.07  ActiveDisplayYMaximum=0.07  DataLoggingVariableName=v29
      Scope26 settings: ActiveDisplayYMinimum=-0.07  ActiveDisplayYMaximum=0.07  DataLoggingVariableName=v30
      Scope27 settings: ActiveDisplayYMinimum=-0.07  ActiveDisplayYMaximum=0.07  DataLoggingVariableName=v31
      Scope28 settings: ActiveDisplayYMinimum=-0.07  ActiveDisplayYMaximum=0.07  DataLoggingVariableName=v32
      Scope29 settings: ActiveDisplayYMinimum=-0.07  ActiveDisplayYMaximum=0.07  DataLoggingVariableName=v47
      Scope3 settings: ActiveDisplayYMinimum=-0.07  ActiveDisplayYMaximum=0.07  DataLoggingVariableName=v34
      Scope37 settings: ActiveDisplayYMinimum=-0.07  ActiveDisplayYMaximum=0.07  DataLoggingVariableName=v58
      Scope38 settings: ActiveDisplayYMinimum=-0.07  ActiveDisplayYMaximum=0.07  DataLoggingVariableName=v52
      Scope39 settings: ActiveDisplayYMinimum=-0.07  ActiveDisplayYMaximum=0.07  DataLoggingVariableName=v53
      Scope4 settings: ActiveDisplayYMinimum=-0.07  ActiveDisplayYMaximum=0.07  DataLoggingVariableName=v35
      Scope40 settings: ActiveDisplayYMinimum=-0.07  ActiveDisplayYMaximum=0.07  DataLoggingVariableName=v54
      Scope41 settings: ActiveDisplayYMinimum=-0.07  ActiveDisplayYMaximum=0.07  DataLoggingVariableName=v55
      Scope42 settings: ActiveDisplayYMinimum=-0.07  ActiveDisplayYMaximum=0.07  DataLoggingVariableName=v56
      Scope43 settings: ActiveDisplayYMinimum=-0.07  ActiveDisplayYMaximum=0.07  DataLoggingVariableName=v57
      Scope45 settings: ActiveDisplayYMinimum=-0.07  ActiveDisplayYMaximum=0.07  DataLoggingVariableName=v59
      Scope46 settings: ActiveDisplayYMinimum=-0.07  ActiveDisplayYMaximum=0.07  DataLoggingVariableName=v60
      Scope47 settings: ActiveDisplayYMinimum=-0.07  ActiveDisplayYMaximum=0.07  DataLoggingVariableName=v61
      Scope48 settings: ActiveDisplayYMinimum=-0.07  ActiveDisplayYMaximum=0.07  DataLoggingVariableName=v73
      Scope49 settings: ActiveDisplayYMinimum=-0.07  ActiveDisplayYMaximum=0.07  DataLoggingVariableName=v76
      Scope5 settings: ActiveDisplayYMinimum=-0.07  ActiveDisplayYMaximum=0.07  DataLoggingVariableName=v36
      Scope6 settings: ActiveDisplayYMinimum=-0.07  ActiveDisplayYMaximum=0.07  DataLoggingVariableName=v37
      Scope7 settings: ActiveDisplayYMinimum=-0.07  ActiveDisplayYMaximum=0.07  DataLoggingVariableName=v26
      Scope8 settings: ActiveDisplayYMinimum=-0.07  ActiveDisplayYMaximum=0.07  DataLoggingVariableName=v7
      Scope9 settings: ActiveDisplayYMinimum=-0.07  ActiveDisplayYMaximum=0.07  DataLoggingVariableName=v38
  W1 : ToWorkspace  VariableName=Qe  SampleTime=1/60
  W2 : ToWorkspace  VariableName=Pe  SampleTime=1/60
  W3 : ToWorkspace  VariableName=Vt  SampleTime=1/60
  W4 : ToWorkspace  VariableName=EFD  SampleTime=1/60
  W_gens : Mux  Inputs=10
  W_gens1 : Mux  Inputs=10
  W_gens2 : Mux  Inputs=10
  W_gens3 : Mux  Inputs=9
  wires:
  [Pe3] -> W_gens/3, Scope7/1
  [Pe2] -> W_gens/2, Scope8/1
  [Vt2] -> Complex to Magnitude-Angle39/1
  Complex to Magnitude-Angle39/1 -> Scope43/1, W_gens2/2
  [Vt3] -> Complex to Magnitude-Angle40/1
  Complex to Magnitude-Angle40/1 -> Scope38/1, W_gens2/3
  [Vt4] -> Complex to Magnitude-Angle41/1
  Complex to Magnitude-Angle41/1 -> Scope39/1, W_gens2/4
  [Vt5] -> Complex to Magnitude-Angle42/1
  Complex to Magnitude-Angle42/1 -> Scope40/1, W_gens2/5
  [Vt6] -> Complex to Magnitude-Angle43/1
  Complex to Magnitude-Angle43/1 -> W_gens2/6, Scope41/1
  [Vt7] -> Complex to Magnitude-Angle44/1
  Complex to Magnitude-Angle44/1 -> Scope42/1, W_gens2/7
  [Vt8] -> Complex to Magnitude-Angle45/1
  Complex to Magnitude-Angle45/1 -> Scope45/1, W_gens2/8
  [Vt9] -> Complex to Magnitude-Angle46/1
  Complex to Magnitude-Angle46/1 -> W_gens2/9, Scope46/1
  [Pe6] -> W_gens/6, Scope25/1
  [Pe5] -> W_gens/5, Scope26/1
  [Pe7] -> W_gens/7, Scope24/1
  [Pe9] -> W_gens/9, Scope28/1
  [Pe8] -> W_gens/8, Scope29/1
  [Pe10] -> W_gens/10, Scope27/1
  [Q3] -> W_gens1/3, Scope11/1
  [Q2] -> W_gens1/2, Scope12/1
  [Q4] -> W_gens1/4, Scope1/1
  [Q6] -> W_gens1/6, Scope3/1
  [Q5] -> W_gens1/5, Scope4/1
  [Q7] -> W_gens1/7, Scope2/1
  [Q9] -> W_gens1/9, Scope6/1
  [Q8] -> W_gens1/8, Scope9/1
  [Q10] -> W_gens1/10, Scope5/1
  [EFD2] -> W_gens3/2, Scope18/1
  [EFD3] -> Scope13/1, W_gens3/3
  [EFD4] -> W_gens3/4, Scope14/1
  [EFD5] -> W_gens3/5, Scope15/1
  [EFD6] -> W_gens3/6, Scope16/1
  [EFD7] -> W_gens3/7, Scope17/1
  [EFD8] -> W_gens3/8, Scope20/1
  [EFD9] -> Scope21/1, W_gens3/9
  [Pe4] -> W_gens/4, Scope10/1
  [Pe1] -> W_gens/1, Scope49/1
  Complex to Magnitude-Angle1/1 -> W_gens2/1, Scope48/1
  [Q1] -> W_gens1/1, Scope37/1
  [EFD1] -> W_gens3/1, Scope47/1
  [Vt1] -> Complex to Magnitude-Angle1/1
  W_gens/1 -> W2/1
  W_gens1/1 -> W1/1
  W_gens2/1 -> W3/1
  W_gens3/1 -> W4/1

== system NE39bus_modified/System Data ==
  ->pu : Gain  Gain=1/(230e3/sqrt(3)*sqrt(2))  SaturateOnIntegerOverflow=on  OutDataTypeStr=Inherit: Same as input  ParamDataTypeStr=Inherit: Same as input
  3-Phase Active & Reactive Power (Phasor Type) : powerlib_extras/Phasor Library/3-Phase Active & Reactive Power (Phasor Type)
  Complex to Magnitude-Angle : ComplexToMagnitudeAngle  Output=Magnitude
  Complex to Magnitude-Angle1 : ComplexToMagnitudeAngle  Output=Magnitude
  Mux : Mux  Inputs=2
  P34 : Gain  Gain=1e-6  SaturateOnIntegerOverflow=on  OutDataTypeStr=Inherit: Same as input  ParamDataTypeStr=Inherit: Same as input
  Selector : Selector  InputPortWidth=2  IndexOptions=Index vector (dialog)  Indices=1  OutputSizes=1
  Sequence Analyzer (Phasor Type) : powerlib_extras/Phasor Library/Sequence Analyzer (Phasor Type)  seq=Positive
  Sequence Analyzer (Phasor Type)1 : powerlib_extras/Phasor Library/Sequence Analyzer (Phasor Type)  seq=Positive
  Terminator1 : Terminator
  Terminator2 : Terminator
  Vabc_B3 : Scope
      settings: TimeSpan=10  ActiveDisplayYMinimum=20  ActiveDisplayYMaximum=90  DataLoggingVariableName=mach3
  Vabc_B4 : Scope
      settings: TimeSpan=10  ActiveDisplayYMinimum=20  ActiveDisplayYMaximum=90  DataLoggingVariableName=mach2
  W2 : ToWorkspace  VariableName=P21  SampleTime=1/60
  Vps : Outport
  p34 : Outport  Port=2
  wires:
  [Vabc_B4] -> Sequence Analyzer (Phasor Type)/1, 3-Phase Active & Reactive Power (Phasor Type)/1, Complex to Magnitude-Angle/1
  [Vabc_B3] -> Sequence Analyzer (Phasor Type)1/1, Complex to Magnitude-Angle1/1
  Sequence Analyzer (Phasor Type)/2 -> Terminator1/1
  Sequence Analyzer (Phasor Type)1/2 -> Terminator2/1
  Sequence Analyzer (Phasor Type)1/1 -> Mux/2
  [Iabc_B4] -> 3-Phase Active & Reactive Power (Phasor Type)/2
  3-Phase Active & Reactive Power (Phasor Type)/1 -> Selector/1
  ->pu/1 -> Vps/1
  Sequence Analyzer (Phasor Type)/1 -> Mux/1
  Mux/1 -> ->pu/1
  P34/1 -> p34/1, W2/1
  Complex to Magnitude-Angle/1 -> Vabc_B4/1
  Complex to Magnitude-Angle1/1 -> Vabc_B3/1
  Selector/1 -> P34/1

== system NE39bus_modified/VSG_ES1 ==
  omega_ref : Inport
  delta_M : Inport  Port=2
  delta_D : Inport  Port=3
  P_ref : Inport  Port=4
  P_e : Inport  Port=5
  D0 : Constant  Value=3
  Div_M : Product  Inputs=*/
  Int_delta : Integrator
  Int_omega : Integrator  InitialCondition=1.0  LimitOutput=on  UpperSaturationLimit=1.1  LowerSaturationLimit=0.9
  M0 : Constant  Value=12
  One : Constant  Value=1.0
  Prod_D : Product  Inputs=**
  Sat_D : Saturate  UpperLimit=7.5  LowerLimit=1.5
  Sat_M : Saturate  UpperLimit=30  LowerLimit=6
  Sum_D : Sum
  Sum_M : Sum
  Sum_P : Sum  Inputs=+--
  Sum_dev : Sum  Inputs=+-
  omega_err : Sum  Inputs=+-
  omega_n : Gain  Gain=314.1593
  omega : Outport
  delta : Outport  Port=2
  P_out : Outport  Port=3
  wires:
  M0/1 -> Sum_M/1
  delta_M/1 -> Sum_M/2
  Sum_M/1 -> Sat_M/1
  D0/1 -> Sum_D/1
  delta_D/1 -> Sum_D/2
  Sum_D/1 -> Sat_D/1
  Sat_D/1 -> Prod_D/1
  omega_err/1 -> Prod_D/2
  P_ref/1 -> Sum_P/1
  P_e/1 -> Sum_P/2
  Prod_D/1 -> Sum_P/3
  Sum_P/1 -> Div_M/1, P_out/1
  Sat_M/1 -> Div_M/2
  Div_M/1 -> Int_omega/1
  Int_omega/1 -> omega_err/1, Sum_dev/1, omega/1
  omega_ref/1 -> omega_err/2
  One/1 -> Sum_dev/2
  Sum_dev/1 -> omega_n/1
  omega_n/1 -> Int_delta/1
  Int_delta/1 -> delta/1

== system NE39bus_modified/VSG_ES2 ==
  omega_ref : Inport
  delta_M : Inport  Port=2
  delta_D : Inport  Port=3
  P_ref : Inport  Port=4
  P_e : Inport  Port=5
  D0 : Constant  Value=3
  Div_M : Product  Inputs=*/
  Int_delta : Integrator
  Int_omega : Integrator  InitialCondition=1.0  LimitOutput=on  UpperSaturationLimit=1.1  LowerSaturationLimit=0.9
  M0 : Constant  Value=12
  One : Constant  Value=1.0
  Prod_D : Product  Inputs=**
  Sat_D : Saturate  UpperLimit=7.5  LowerLimit=1.5
  Sat_M : Saturate  UpperLimit=30  LowerLimit=6
  Sum_D : Sum
  Sum_M : Sum
  Sum_P : Sum  Inputs=+--
  Sum_dev : Sum  Inputs=+-
  omega_err : Sum  Inputs=+-
  omega_n : Gain  Gain=314.1593
  omega : Outport
  delta : Outport  Port=2
  P_out : Outport  Port=3
  wires:
  M0/1 -> Sum_M/1
  delta_M/1 -> Sum_M/2
  Sum_M/1 -> Sat_M/1
  D0/1 -> Sum_D/1
  delta_D/1 -> Sum_D/2
  Sum_D/1 -> Sat_D/1
  Sat_D/1 -> Prod_D/1
  omega_err/1 -> Prod_D/2
  P_ref/1 -> Sum_P/1
  P_e/1 -> Sum_P/2
  Prod_D/1 -> Sum_P/3
  Sum_P/1 -> Div_M/1, P_out/1
  Sat_M/1 -> Div_M/2
  Div_M/1 -> Int_omega/1
  Int_omega/1 -> omega_err/1, Sum_dev/1, omega/1
  omega_ref/1 -> omega_err/2
  One/1 -> Sum_dev/2
  Sum_dev/1 -> omega_n/1
  omega_n/1 -> Int_delta/1
  Int_delta/1 -> delta/1

== system NE39bus_modified/VSG_ES3 ==
  omega_ref : Inport
  delta_M : Inport  Port=2
  delta_D : Inport  Port=3
  P_ref : Inport  Port=4
  P_e : Inport  Port=5
  D0 : Constant  Value=3
  Div_M : Product  Inputs=*/
  Int_delta : Integrator
  Int_omega : Integrator  InitialCondition=1.0  LimitOutput=on  UpperSaturationLimit=1.1  LowerSaturationLimit=0.9
  M0 : Constant  Value=12
  One : Constant  Value=1.0
  Prod_D : Product  Inputs=**
  Sat_D : Saturate  UpperLimit=7.5  LowerLimit=1.5
  Sat_M : Saturate  UpperLimit=30  LowerLimit=6
  Sum_D : Sum
  Sum_M : Sum
  Sum_P : Sum  Inputs=+--
  Sum_dev : Sum  Inputs=+-
  omega_err : Sum  Inputs=+-
  omega_n : Gain  Gain=314.1593
  omega : Outport
  delta : Outport  Port=2
  P_out : Outport  Port=3
  wires:
  M0/1 -> Sum_M/1
  delta_M/1 -> Sum_M/2
  Sum_M/1 -> Sat_M/1
  D0/1 -> Sum_D/1
  delta_D/1 -> Sum_D/2
  Sum_D/1 -> Sat_D/1
  Sat_D/1 -> Prod_D/1
  omega_err/1 -> Prod_D/2
  P_ref/1 -> Sum_P/1
  P_e/1 -> Sum_P/2
  Prod_D/1 -> Sum_P/3
  Sum_P/1 -> Div_M/1, P_out/1
  Sat_M/1 -> Div_M/2
  Div_M/1 -> Int_omega/1
  Int_omega/1 -> omega_err/1, Sum_dev/1, omega/1
  omega_ref/1 -> omega_err/2
  One/1 -> Sum_dev/2
  Sum_dev/1 -> omega_n/1
  omega_n/1 -> Int_delta/1
  Int_delta/1 -> delta/1

== system NE39bus_modified/VSG_ES4 ==
  omega_ref : Inport
  delta_M : Inport  Port=2
  delta_D : Inport  Port=3
  P_ref : Inport  Port=4
  P_e : Inport  Port=5
  D0 : Constant  Value=3
  Div_M : Product  Inputs=*/
  Int_delta : Integrator
  Int_omega : Integrator  InitialCondition=1.0  LimitOutput=on  UpperSaturationLimit=1.1  LowerSaturationLimit=0.9
  M0 : Constant  Value=12
  One : Constant  Value=1.0
  Prod_D : Product  Inputs=**
  Sat_D : Saturate  UpperLimit=7.5  LowerLimit=1.5
  Sat_M : Saturate  UpperLimit=30  LowerLimit=6
  Sum_D : Sum
  Sum_M : Sum
  Sum_P : Sum  Inputs=+--
  Sum_dev : Sum  Inputs=+-
  omega_err : Sum  Inputs=+-
  omega_n : Gain  Gain=314.1593
  omega : Outport
  delta : Outport  Port=2
  P_out : Outport  Port=3
  wires:
  M0/1 -> Sum_M/1
  delta_M/1 -> Sum_M/2
  Sum_M/1 -> Sat_M/1
  D0/1 -> Sum_D/1
  delta_D/1 -> Sum_D/2
  Sum_D/1 -> Sat_D/1
  Sat_D/1 -> Prod_D/1
  omega_err/1 -> Prod_D/2
  P_ref/1 -> Sum_P/1
  P_e/1 -> Sum_P/2
  Prod_D/1 -> Sum_P/3
  Sum_P/1 -> Div_M/1, P_out/1
  Sat_M/1 -> Div_M/2
  Div_M/1 -> Int_omega/1
  Int_omega/1 -> omega_err/1, Sum_dev/1, omega/1
  omega_ref/1 -> omega_err/2
  One/1 -> Sum_dev/2
  Sum_dev/1 -> omega_n/1
  omega_n/1 -> Int_delta/1
  Int_delta/1 -> delta/1

== system NE39bus_modified/VSG_ES5 ==
  omega_ref : Inport
  delta_M : Inport  Port=2
  delta_D : Inport  Port=3
  P_ref : Inport  Port=4
  P_e : Inport  Port=5
  D0 : Constant  Value=3
  Div_M : Product  Inputs=*/
  Int_delta : Integrator
  Int_omega : Integrator  InitialCondition=1.0  LimitOutput=on  UpperSaturationLimit=1.1  LowerSaturationLimit=0.9
  M0 : Constant  Value=12
  One : Constant  Value=1.0
  Prod_D : Product  Inputs=**
  Sat_D : Saturate  UpperLimit=7.5  LowerLimit=1.5
  Sat_M : Saturate  UpperLimit=30  LowerLimit=6
  Sum_D : Sum
  Sum_M : Sum
  Sum_P : Sum  Inputs=+--
  Sum_dev : Sum  Inputs=+-
  omega_err : Sum  Inputs=+-
  omega_n : Gain  Gain=314.1593
  omega : Outport
  delta : Outport  Port=2
  P_out : Outport  Port=3
  wires:
  M0/1 -> Sum_M/1
  delta_M/1 -> Sum_M/2
  Sum_M/1 -> Sat_M/1
  D0/1 -> Sum_D/1
  delta_D/1 -> Sum_D/2
  Sum_D/1 -> Sat_D/1
  Sat_D/1 -> Prod_D/1
  omega_err/1 -> Prod_D/2
  P_ref/1 -> Sum_P/1
  P_e/1 -> Sum_P/2
  Prod_D/1 -> Sum_P/3
  Sum_P/1 -> Div_M/1, P_out/1
  Sat_M/1 -> Div_M/2
  Div_M/1 -> Int_omega/1
  Int_omega/1 -> omega_err/1, Sum_dev/1, omega/1
  omega_ref/1 -> omega_err/2
  One/1 -> Sum_dev/2
  Sum_dev/1 -> omega_n/1
  omega_n/1 -> Int_delta/1
  Int_delta/1 -> delta/1

== system NE39bus_modified/VSG_ES6 ==
  omega_ref : Inport
  delta_M : Inport  Port=2
  delta_D : Inport  Port=3
  P_ref : Inport  Port=4
  P_e : Inport  Port=5
  D0 : Constant  Value=3
  Div_M : Product  Inputs=*/
  Int_delta : Integrator
  Int_omega : Integrator  InitialCondition=1.0  LimitOutput=on  UpperSaturationLimit=1.1  LowerSaturationLimit=0.9
  M0 : Constant  Value=12
  One : Constant  Value=1.0
  Prod_D : Product  Inputs=**
  Sat_D : Saturate  UpperLimit=7.5  LowerLimit=1.5
  Sat_M : Saturate  UpperLimit=30  LowerLimit=6
  Sum_D : Sum
  Sum_M : Sum
  Sum_P : Sum  Inputs=+--
  Sum_dev : Sum  Inputs=+-
  omega_err : Sum  Inputs=+-
  omega_n : Gain  Gain=314.1593
  omega : Outport
  delta : Outport  Port=2
  P_out : Outport  Port=3
  wires:
  M0/1 -> Sum_M/1
  delta_M/1 -> Sum_M/2
  Sum_M/1 -> Sat_M/1
  D0/1 -> Sum_D/1
  delta_D/1 -> Sum_D/2
  Sum_D/1 -> Sat_D/1
  Sat_D/1 -> Prod_D/1
  omega_err/1 -> Prod_D/2
  P_ref/1 -> Sum_P/1
  P_e/1 -> Sum_P/2
  Prod_D/1 -> Sum_P/3
  Sum_P/1 -> Div_M/1, P_out/1
  Sat_M/1 -> Div_M/2
  Div_M/1 -> Int_omega/1
  Int_omega/1 -> omega_err/1, Sum_dev/1, omega/1
  omega_ref/1 -> omega_err/2
  One/1 -> Sum_dev/2
  Sum_dev/1 -> omega_n/1
  omega_n/1 -> Int_delta/1
  Int_delta/1 -> delta/1

== system NE39bus_modified/VSG_ES7 ==
  omega_ref : Inport
  delta_M : Inport  Port=2
  delta_D : Inport  Port=3
  P_ref : Inport  Port=4
  P_e : Inport  Port=5
  D0 : Constant  Value=3
  Div_M : Product  Inputs=*/
  Int_delta : Integrator
  Int_omega : Integrator  InitialCondition=1.0  LimitOutput=on  UpperSaturationLimit=1.1  LowerSaturationLimit=0.9
  M0 : Constant  Value=12
  One : Constant  Value=1.0
  Prod_D : Product  Inputs=**
  Sat_D : Saturate  UpperLimit=7.5  LowerLimit=1.5
  Sat_M : Saturate  UpperLimit=30  LowerLimit=6
  Sum_D : Sum
  Sum_M : Sum
  Sum_P : Sum  Inputs=+--
  Sum_dev : Sum  Inputs=+-
  omega_err : Sum  Inputs=+-
  omega_n : Gain  Gain=314.1593
  omega : Outport
  delta : Outport  Port=2
  P_out : Outport  Port=3
  wires:
  M0/1 -> Sum_M/1
  delta_M/1 -> Sum_M/2
  Sum_M/1 -> Sat_M/1
  D0/1 -> Sum_D/1
  delta_D/1 -> Sum_D/2
  Sum_D/1 -> Sat_D/1
  Sat_D/1 -> Prod_D/1
  omega_err/1 -> Prod_D/2
  P_ref/1 -> Sum_P/1
  P_e/1 -> Sum_P/2
  Prod_D/1 -> Sum_P/3
  Sum_P/1 -> Div_M/1, P_out/1
  Sat_M/1 -> Div_M/2
  Div_M/1 -> Int_omega/1
  Int_omega/1 -> omega_err/1, Sum_dev/1, omega/1
  omega_ref/1 -> omega_err/2
  One/1 -> Sum_dev/2
  Sum_dev/1 -> omega_n/1
  omega_n/1 -> Int_delta/1
  Int_delta/1 -> delta/1

== system NE39bus_modified/VSG_ES8 ==
  omega_ref : Inport
  delta_M : Inport  Port=2
  delta_D : Inport  Port=3
  P_ref : Inport  Port=4
  P_e : Inport  Port=5
  D0 : Constant  Value=3
  Div_M : Product  Inputs=*/
  Int_delta : Integrator
  Int_omega : Integrator  InitialCondition=1.0  LimitOutput=on  UpperSaturationLimit=1.1  LowerSaturationLimit=0.9
  M0 : Constant  Value=12
  One : Constant  Value=1.0
  Prod_D : Product  Inputs=**
  Sat_D : Saturate  UpperLimit=7.5  LowerLimit=1.5
  Sat_M : Saturate  UpperLimit=30  LowerLimit=6
  Sum_D : Sum
  Sum_M : Sum
  Sum_P : Sum  Inputs=+--
  Sum_dev : Sum  Inputs=+-
  omega_err : Sum  Inputs=+-
  omega_n : Gain  Gain=314.1593
  omega : Outport
  delta : Outport  Port=2
  P_out : Outport  Port=3
  wires:
  M0/1 -> Sum_M/1
  delta_M/1 -> Sum_M/2
  Sum_M/1 -> Sat_M/1
  D0/1 -> Sum_D/1
  delta_D/1 -> Sum_D/2
  Sum_D/1 -> Sat_D/1
  Sat_D/1 -> Prod_D/1
  omega_err/1 -> Prod_D/2
  P_ref/1 -> Sum_P/1
  P_e/1 -> Sum_P/2
  Prod_D/1 -> Sum_P/3
  Sum_P/1 -> Div_M/1, P_out/1
  Sat_M/1 -> Div_M/2
  Div_M/1 -> Int_omega/1
  Int_omega/1 -> omega_err/1, Sum_dev/1, omega/1
  omega_ref/1 -> omega_err/2
  One/1 -> Sum_dev/2
  Sum_dev/1 -> omega_n/1
  omega_n/1 -> Int_delta/1
  Int_delta/1 -> delta/1
